simulink model "tps_pwm_curve"  (R2023a)
settings: Solver=ode3  StartTime=0.0  StopTime=200  RelTol=1e-3  EnableMultiTasking=on
libraries: arduinolib x3, arduinosensorlib x1
settings Model: ExtModeTrigDuration=2  Creator=zapat  LastModifiedBy=zapat
settings SolverCC: AlgebraicLoopSolver=TrustRegion
settings DataIOCC: LimitDataPoints=on  SaveFormat=Array
settings OptimizationCC: ExpressionDepthLimit=2147483647  LifeSpan=Inf  MaxStackSize=64
settings DebuggingCC: UnderspecifiedInitializationDetection=Classic  MergeDetectMultiDrivingBlocksExec=none  FcnCallInpInsideContextMsg=warning  UnconnectedInputMsg=warning  UnconnectedOutputMsg=warning  UnconnectedLineMsg=warning  AllowSymbolicDim=off  StateNameClashWarn=warning  SFUnexpectedBacktrackingDiag=warning  SFNoUnconditionalDefaultTransitionDiag=warning  SFExecutionAtInitializationDiag=none  ArithmeticOperatorsInVariantConditions=warning
settings HardwareCC: ProdBitPerPointer=32  ProdBitPerSizeT=32  ProdBitPerPtrDiffT=32  ProdLargestAtomicInteger=Long  ProdLargestAtomicFloat=Double  ProdWordSize=32  ProdHWDeviceType=ARM Compatible->ARM Cortex  UseEmbeddedCoderFeatures=off  UseSimulinkCoderFeatures=off
settings ModelReferenceCC: EnableRefExpFcnMdlSchedulingChecks=on  PropagateSignalLabelsOutOfModel=off
settings SFSimCC: SimUseLocalCustomCode=off  CustomCodeUndefinedFunction=UseInterfaceOnly
settings RTWCC: Description=Embedded Coder  SystemTargetFile=ert.tlc  HardwareBoard=ESP32-WROOM(Arduino Compatible)  TemplateMakefile=ert_default_tmf  RTWVerbose=off  RTWUseLocalCustomCode=off  Toolchain=ESP32  BuildConfiguration=Faster Runs
settings CodeAppCC: ForceParamTrailComments=on  OperatorAnnotations=on  StateflowObjectComments=on  MATLABSourceComments=on
settings ERTTargetCC: MultiwordLength=2048  ERTCustomFileBanners=off  SupportContinuousTime=on  SupportNonInlinedSFcns=on  RemoveResetFunc=off  SupportVariableSizeSignals=on  ModelStepFunctionPrototypeControlCompliant=off  ExtModeTransport=3  ExtModeStaticAlloc=on  ExtModeAutomaticAllocSize=off  ExtModeStaticAllocSize=65536  ExtModeMexFile=ext_xcp  ExtModeIntrfLevel=Level2 - Open  ERTSrcFileBannerTemplate=codertarget_code_template.cgt  ERTHdrFileBannerTemplate=codertarget_code_template.cgt  ERTDataSrcFileTemplate=codertarget_code_template.cgt  ERTDataHdrFileTemplate=codertarget_code_template.cgt
settings ConfigComp: CovMetricSettings=dw  CovSaveCumulativeToWorkspaceVar=on  CovSaveSingleToWorkspaceVar=on  CovExternalEMLEnable=off  CovSFcnEnable=off

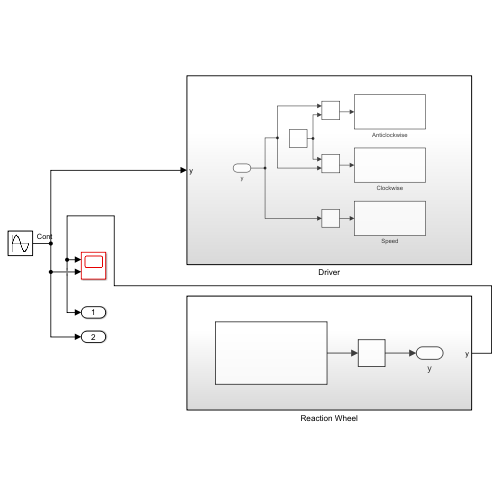
[thumbnail: Simulink's stored preview of the top-level diagram]
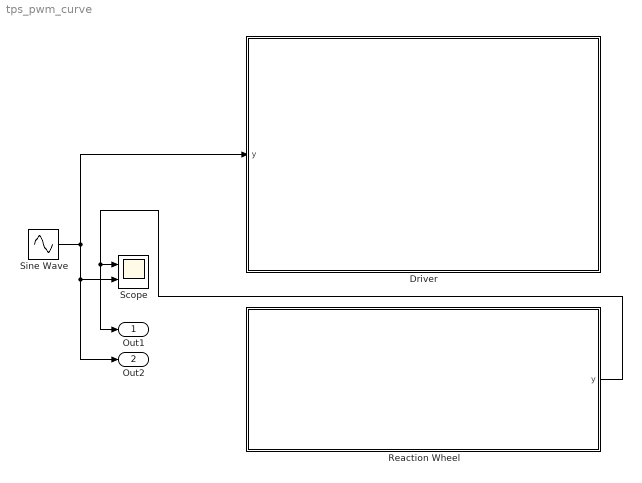
== system tps_pwm_curve ==
  Driver : Subsystem
  Reaction Wheel : Subsystem
  Scope : Scope  NumInputPorts=2
  Sine Wave : Sin  Amplitude=255  Frequency=2*pi/200  SampleTime=0
  Out1 : Outport
  Out2 : Outport  Port=2
  wires:
  Sine Wave/1 -> Driver/1(y), Out2/1, Scope/2
  Reaction Wheel/1(y) -> Out1/1, Scope/1

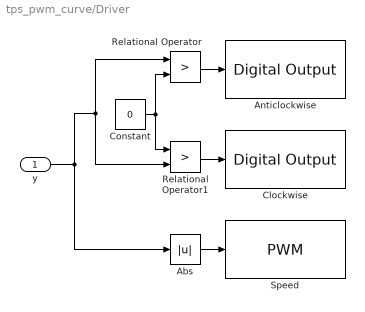
== system tps_pwm_curve/Driver ==
  y : Inport
  Abs : Abs  SaturateOnIntegerOverflow=off
  Anticlockwise : arduinolib/Digital Output  pinNumber=2  Direction=output  blockPlatform=arduino
  Clockwise : arduinolib/Digital Output  pinNumber=0  Direction=output  blockPlatform=arduino
  Constant : Constant  Value=0
  Relational Operator : RelationalOperator  Operator=>  OutDataTypeStr=boolean  RndMeth=Simplest  InputSameDT=off
  Relational Operator1 : RelationalOperator  Operator=>  OutDataTypeStr=boolean  RndMeth=Simplest  InputSameDT=off
  Speed : arduinolib/PWM  pinNumber=15  frequencyType=Default  desiredFrequency=490.2  achievableFrequency=490.2
  wires:
  Relational Operator/1 -> Anticlockwise/1
  y/1 -> Abs/1, Relational Operator1/2, Relational Operator/1
  Constant/1 -> Relational Operator/2, Relational Operator1/1
  Relational Operator1/1 -> Clockwise/1
  Abs/1 -> Speed/1

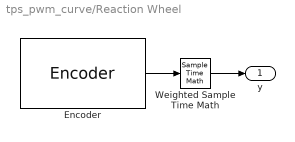
== system tps_pwm_curve/Reaction Wheel ==
  Encoder : arduinosensorlib/Encoder  InputA=4  InputB=16  Mode=Reset at each Sample time  SampleTime=-1
  Weighted Sample Time Math : SampleTimeMath  TsampMathOp=/
  y : Outport
  wires:
  Encoder/1 -> Weighted Sample Time Math/1
  Weighted Sample Time Math/1 -> y/1
